simulink model "powerwindow_sl_v01"  (R2020a)
settings: Solver=ode1  StartTime=0.0  StopTime=20.0  FixedStep=0.01  RelTol=1e-3
undefined symbols (not defined in the file): auto_down_time, auto_up_time, emergency_down_time, position_endstop_top
settings Model: TunableVars=auto_down_time,auto_up_time,emergency_down_time,position_endstop_top  TunableVarsStorageClass=Auto,Auto,Auto,Auto  TunableVarsTypeQualifier=,,,  Creator=Wolfgang Meincke  LastModifiedBy=wolfgangmeincke
settings DataIOCC: LimitDataPoints=on  SaveFormat=Array  SignalLoggingSaveFormat=ModelDataLogs  ReturnWorkspaceOutputs=off
settings OptimizationCC: BlockReduction=off  BooleanDataType=off  ConditionallyExecuteInputs=off  EnableMemcpy=off  ExpressionDepthLimit=2147483647  ZeroExternalMemoryAtStartup=off  ZeroInternalMemoryAtStartup=off  InitFltsAndDblsToZero=on  NoFixptDivByZeroProtection=on  LifeSpan=1  EfficientTunableParamExpr=on
settings DebuggingCC: RTPrefix=none  SaveWithParameterizedLinksMsg=none  UnderspecifiedInitializationDetection=Classic  MergeDetectMultiDrivingBlocksExec=none  MultiTaskDSMMsg=warning  MultiTaskCondExecSysMsg=none  ParameterPrecisionLossMsg=none  FcnCallInpInsideContextMsg=warning  UnconnectedInputMsg=none  UnconnectedOutputMsg=none  StateNameClashWarn=warning  SFUnexpectedBacktrackingDiag=warning  SFNoUnconditionalDefaultTransitionDiag=warning  SFExecutionAtInitializationDiag=none  ArithmeticOperatorsInVariantConditions=warning
settings HardwareCC: ProdBitPerPointer=32  ProdBitPerSizeT=32  ProdBitPerPtrDiffT=32  ProdLargestAtomicFloat=None  ProdIntDivRoundTo=Undefined  ProdEndianess=Unspecified  ProdWordSize=32  ProdHWDeviceType=32-bit Generic
settings ModelReferenceCC: PropagateSignalLabelsOutOfModel=off
settings SFSimCC: SimUseLocalCustomCode=off  SimParseCustomCode=off  MATLABDynamicMemAlloc=off  CustomCodeUndefinedFunction=UseInterfaceOnly
settings RTWCC: SystemTargetFile=ert.tlc  GenCodeOnly=on  TemplateMakefile=ert_default_tmf  RTWUseLocalCustomCode=off
settings CodeAppCC: IgnoreCustomStorageClasses=off  ParamNamingRule=LowerCase  StateflowObjectComments=on  InternalIdentifier=Classic
settings ERTTargetCC: MultiwordLength=2048  IncludeMdlTerminateFcn=off  CombineSignalStateStructs=on  SupportAbsoluteTime=off  LogVarNameModifier=_rt  SupportNonFinite=off  SupportComplex=off  RemoveResetFunc=off  ERTCustomFileTemplate=example_file_process.tlc  ConvertIfToSwitch=off  SuppressUnreachableDefaultCases=off
settings ConfigComp: CovMetricSettings=dw  CovSaveCumulativeToWorkspaceVar=on  CovSaveSingleToWorkspaceVar=on  CovExternalEMLEnable=off

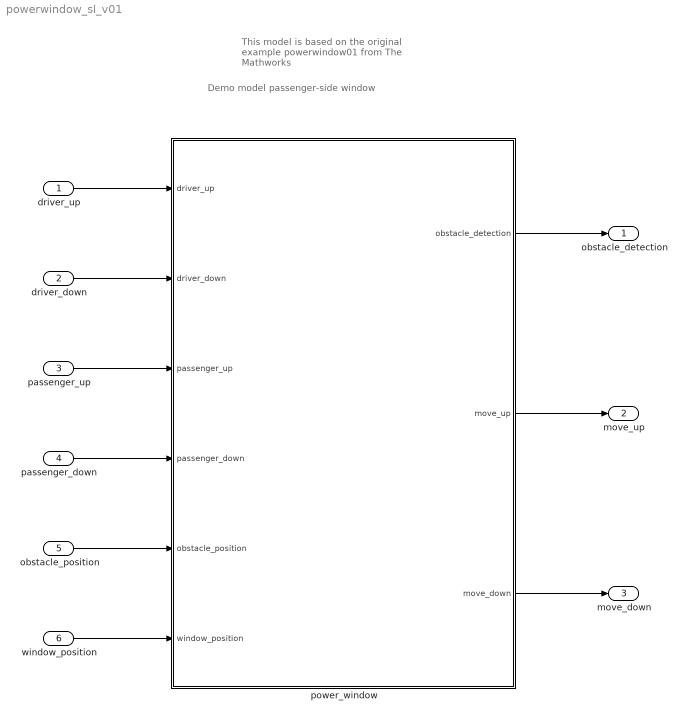
== system powerwindow_sl_v01 ==
  note: Demo model passenger-side window
  note: This model is based on the
      | original example powerwindow01
      | from The Mathworks
  driver_up : Inport  RequirementInfo={} %GIDa_c35cf34b_45f5_487d_8434_6977e2d5d2f3  OutMin=0  OutMax=1  OutDataTypeStr=boolean  PortDimensions=1
  driver_down : Inport  RequirementInfo={} %GIDa_825829a4_4c67_4036_abe4_d775b7ffbdb6  Port=2  OutMin=0  OutMax=1  OutDataTypeStr=boolean  PortDimensions=1
  passenger_up : Inport  RequirementInfo={} %GIDa_896a61d0_51a5_427e_b548_01888eb9493f  Port=3  OutMin=0  OutMax=1  OutDataTypeStr=boolean  PortDimensions=1
  passenger_down : Inport  RequirementInfo={} %GIDa_acad868a_9832_4517_80f1_eb2c424aca82  Port=4  OutMin=0  OutMax=1  OutDataTypeStr=boolean  PortDimensions=1
  obstacle_position : Inport  RequirementInfo={} %GIDa_5be180b3_640c_44df_b132_7c12c9dd4782  Port=5  OutMin=0  OutMax=0.45  OutDataTypeStr=double  PortDimensions=1
  window_position : Inport  RequirementInfo={} %GIDa_279514cf_fecf_4861_97d0_86738c273b33  Port=6  OutMin=0  OutMax=0.45  OutDataTypeStr=double  PortDimensions=1
  power_window : Subsystem
  obstacle_detection : Outport  RequirementInfo={} %GIDa_4eefd6fd_6a0d_4232_ac82_ccb47f3c36e3  OutMin=0  OutMax=1  OutDataTypeStr=boolean  PortDimensions=1
  move_up : Outport  RequirementInfo={} %GIDa_cfaa6890_1b09_43c8_9181_c9775bd2e746  Port=2  OutMin=0  OutMax=1  OutDataTypeStr=boolean  PortDimensions=1
  move_down : Outport  RequirementInfo={} %GIDa_e72b7e0a_8232_4793_901f_580fad4f0530  Port=3  OutMin=0  OutMax=1  OutDataTypeStr=boolean  PortDimensions=1
  wires:
  power_window/3(move_down) -> move_down/1
  power_window/1(obstacle_detection) -> obstacle_detection/1
  window_position/1 -> power_window/6(window_position)
  power_window/2(move_up) -> move_up/1
  driver_up/1 -> power_window/1(driver_up)
  passenger_up/1 -> power_window/3(passenger_up)
  passenger_down/1 -> power_window/4(passenger_down)
  driver_down/1 -> power_window/2(driver_down)
  obstacle_position/1 -> power_window/5(obstacle_position)

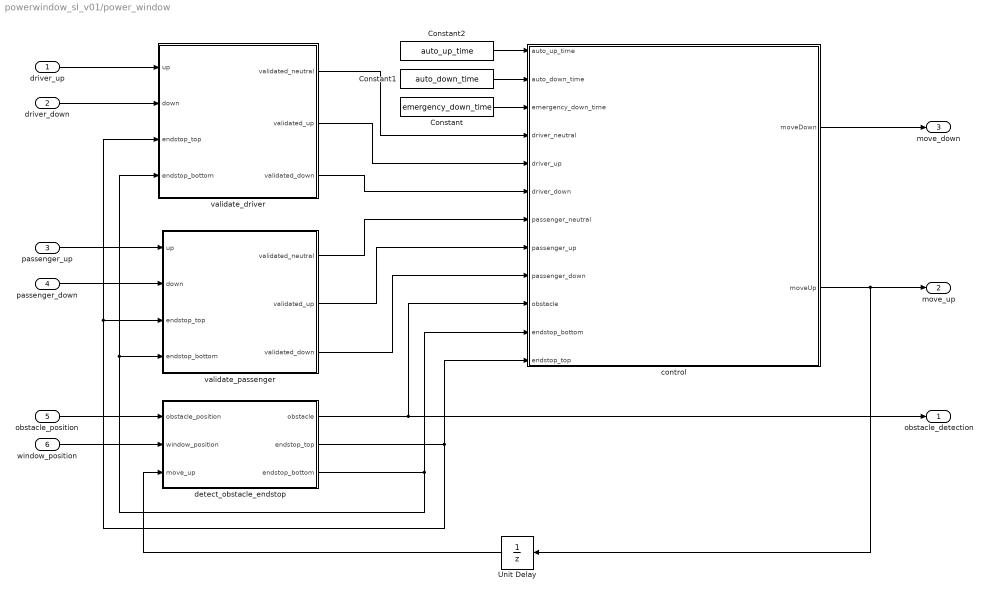
== system powerwindow_sl_v01/power_window ==
  driver_up : Inport  RequirementInfo={} %GIDa_c35cf34b_45f5_487d_8434_6977e2d5d2f3  OutMin=0  OutMax=1  OutDataTypeStr=boolean  PortDimensions=1
  driver_down : Inport  RequirementInfo={} %GIDa_825829a4_4c67_4036_abe4_d775b7ffbdb6  Port=2  OutMin=0  OutMax=1  OutDataTypeStr=boolean  PortDimensions=1
  passenger_up : Inport  RequirementInfo={} %GIDa_896a61d0_51a5_427e_b548_01888eb9493f  Port=3  OutMin=0  OutMax=1  OutDataTypeStr=boolean  PortDimensions=1
  passenger_down : Inport  RequirementInfo={} %GIDa_acad868a_9832_4517_80f1_eb2c424aca82  Port=4  OutMin=0  OutMax=1  OutDataTypeStr=boolean  PortDimensions=1
  obstacle_position : Inport  RequirementInfo={} %GIDa_5be180b3_640c_44df_b132_7c12c9dd4782  Port=5  OutMin=0  OutMax=0.45  OutDataTypeStr=double  PortDimensions=1
  window_position : Inport  RequirementInfo={} %GIDa_279514cf_fecf_4861_97d0_86738c273b33  Port=6  OutMin=0  OutMax=0.45  OutDataTypeStr=double  PortDimensions=1
  Constant : Constant  RequirementInfo={} %GIDa_9514aab4_7290_4656_a952_a9cac9bec120  Value=emergency_down_time  OutDataTypeStr=uint8
  Constant1 : Constant  RequirementInfo={} %GIDa_6c74b792_e839_4a12_ac84_86c7d570a533  Value=auto_down_time  OutDataTypeStr=uint8
  Constant2 : Constant  RequirementInfo={} %GIDa_27bbea0c_c5f9_4e52_b093_a1cd3ec1797f  Value=auto_up_time  OutDataTypeStr=uint8
  Unit Delay : UnitDelay  RequirementInfo={} %GIDa_61c3f994_badd_4b85_b577_84166d45c76a  SampleTime=-1
  control : Stateflow chart  RequirementInfo={} %GIDa_03dc6751_b1fa_4801_9ce5_d6a4ecb5c081
  detect_obstacle_endstop : Subsystem  RequirementInfo={} %GIDa_338a624e_935a_458f_b92a_1404c1b9bbb3  TreatAsAtomicUnit=on  RTWFcnName=detect_obstacle_endstop
      settings: RTWFcnNameOpts=User specified  RTWFileNameOpts=Use function name
  validate_driver : Subsystem  RequirementInfo={} %GIDa_ecdb279d_e424_4d89_b641_a52ee121c2a5  TreatAsAtomicUnit=on  RTWFcnName=validate_driver
      settings: RTWFcnNameOpts=Use subsystem name  RTWFileNameOpts=Use function name
  validate_passenger : Subsystem  RequirementInfo={} %GIDa_33b218b3_9db5_4fe6_9638_6b05429d8e58  TreatAsAtomicUnit=on  RTWFcnName=validate_passenger
      settings: RTWFcnNameOpts=User specified  RTWFileNameOpts=Use subsystem name
  obstacle_detection : Outport  RequirementInfo={} %GIDa_4eefd6fd_6a0d_4232_ac82_ccb47f3c36e3  OutMin=0  OutMax=1  OutDataTypeStr=boolean  PortDimensions=1
  move_up : Outport  RequirementInfo={} %GIDa_cfaa6890_1b09_43c8_9181_c9775bd2e746  Port=2  OutMin=0  OutMax=1  OutDataTypeStr=boolean  PortDimensions=1
  move_down : Outport  RequirementInfo={} %GIDa_e72b7e0a_8232_4793_901f_580fad4f0530  Port=3  OutMin=0  OutMax=1  OutDataTypeStr=boolean  PortDimensions=1
  wires:
  validate_passenger/2(validated_up) -> control/8(passenger_up)
  detect_obstacle_endstop/2(endstop_top) -> validate_passenger/3(endstop_top), validate_driver/3(endstop_top), control/12(endstop_top)
  validate_passenger/1(validated_neutral) -> control/7(passenger_neutral)
  detect_obstacle_endstop/1(obstacle) -> obstacle_detection/1, control/10(obstacle)
  control/2(moveUp) -> move_up/1, Unit Delay/1
  Constant/1 -> control/3(emergency_down_time)
  validate_driver/2(validated_up) -> control/5(driver_up)
  obstacle_position/1 -> detect_obstacle_endstop/1(obstacle_position)
  validate_passenger/3(validated_down) -> control/9(passenger_down)
  passenger_up/1 -> validate_passenger/1(up)
  driver_up/1 -> validate_driver/1(up)
  Constant2/1 -> control/1(auto_up_time)
  Constant1/1 -> control/2(auto_down_time)
  window_position/1 -> detect_obstacle_endstop/2(window_position)
  driver_down/1 -> validate_driver/2(down)
  detect_obstacle_endstop/3(endstop_bottom) -> validate_passenger/4(endstop_bottom), validate_driver/4(endstop_bottom), control/11(endstop_bottom)
  validate_driver/3(validated_down) -> control/6(driver_down)
  control/1(moveDown) -> move_down/1
  Unit Delay/1 -> detect_obstacle_endstop/3(move_up)
  validate_driver/1(validated_neutral) -> control/4(driver_neutral)
  passenger_down/1 -> validate_passenger/2(down)

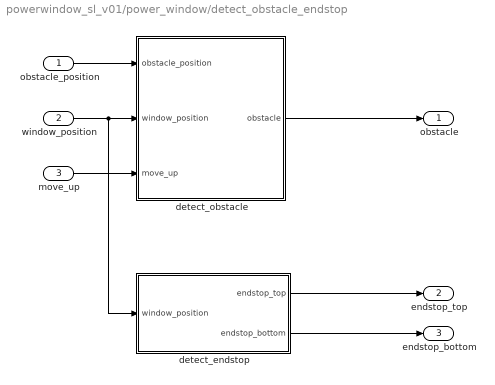
== system powerwindow_sl_v01/power_window/detect_obstacle_endstop ==
  obstacle_position : Inport  RequirementInfo={} %GIDa_129d33c9_dbad_4345_a32e_36abfffa4eb8
  window_position : Inport  RequirementInfo={} %GIDa_0a19a92c_2144_4371_9df6_11f6bf2158cd  Port=2
  move_up : Inport  RequirementInfo={} %GIDa_fb499b4a_e779_426c_9231_7bb7c4693121  Port=3
  detect_endstop : Subsystem  RequirementInfo={} %GIDa_94bbc35b_ebf0_4cc3_8650_bc7180b52bf6
  detect_obstacle : Subsystem  RequirementInfo={} %GIDa_c80b8ad7_641a_45a4_83c2_0d5a6b3dc5a0
  obstacle : Outport  RequirementInfo={} %GIDa_f8cefc1d_8d33_4143_9aaf_e393e35a8988
  endstop_top : Outport  RequirementInfo={} %GIDa_3c0c9233_5a48_409d_ac60_81b669eb4a89  Port=2
  endstop_bottom : Outport  RequirementInfo={} %GIDa_25ef007a_9840_4d98_9cf5_d35ec59ee2ed  Port=3
  wires:
  detect_endstop/2(endstop_bottom) -> endstop_bottom/1
  detect_endstop/1(endstop_top) -> endstop_top/1
  detect_obstacle/1(obstacle) -> obstacle/1
  obstacle_position/1 -> detect_obstacle/1(obstacle_position)
  window_position/1 -> detect_endstop/1(window_position), detect_obstacle/2(window_position)
  move_up/1 -> detect_obstacle/3(move_up)

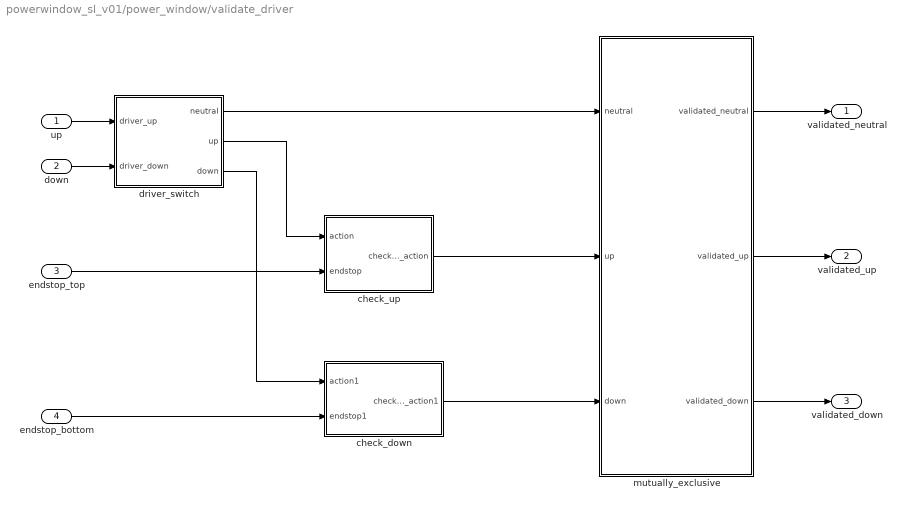
== system powerwindow_sl_v01/power_window/validate_driver ==
  up : Inport  RequirementInfo={} %GIDa_7dda3897_23eb_48f1_9817_08c06aa18141
  down : Inport  RequirementInfo={} %GIDa_9d54edea_1179_4fce_abe2_5db1acfa11b9  Port=2
  endstop_top : Inport  RequirementInfo={} %GIDa_9bd89aaf_7e8b_49dc_b3c1_497d13e079f2  Port=3
  endstop_bottom : Inport  RequirementInfo={} %GIDa_15d013e7_6fa7_49fb_8ea8_038359a3d9b6  Port=4
  check_down : Subsystem  RequirementInfo={} %GIDa_c558df2e_0968_478b_94d3_8b52e729db44
  check_up : Subsystem  RequirementInfo={} %GIDa_680f415b_674f_4667_a838_dd8371ea2197
  driver_switch : Subsystem  RequirementInfo={} %GIDa_e99d5410_be85_4670_8578_fe8e0dfb5d67
  mutually_exclusive : Subsystem  RequirementInfo={} %GIDa_d6baea27_d272_4747_8dc3_6f978df1e0c8
  validated_neutral : Outport  RequirementInfo={} %GIDa_f23c1ed9_f7cc_4416_b545_9bac5c7d020f
  validated_up : Outport  RequirementInfo={} %GIDa_9144ace2_3ce2_4646_bfcc_6ba779b8e848  Port=2
  validated_down : Outport  RequirementInfo={} %GIDa_bb002e94_52f0_4ca7_8c66_58dd2cd42898  Port=3
  wires:
  mutually_exclusive/3(validated_down) -> validated_down/1
  mutually_exclusive/2(validated_up) -> validated_up/1
  mutually_exclusive/1(validated_neutral) -> validated_neutral/1
  check_down/1(checked_action1) -> mutually_exclusive/3(down)
  check_up/1(checked_action) -> mutually_exclusive/2(up)
  driver_switch/1(neutral) -> mutually_exclusive/1(neutral)
  endstop_bottom/1 -> check_down/2(endstop1)
  endstop_top/1 -> check_up/2(endstop)
  driver_switch/3(down) -> check_down/1(action1)
  driver_switch/2(up) -> check_up/1(action)
  down/1 -> driver_switch/2(driver_down)
  up/1 -> driver_switch/1(driver_up)

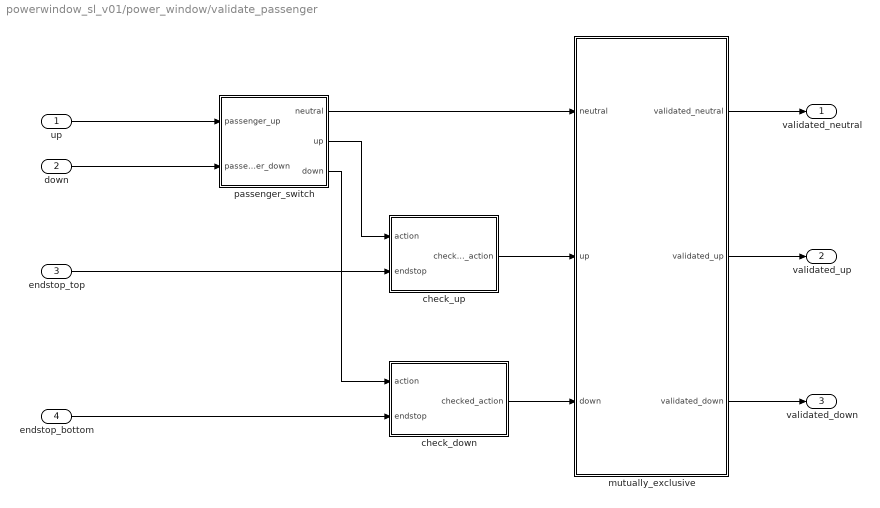
== system powerwindow_sl_v01/power_window/validate_passenger ==
  up : Inport  RequirementInfo={} %GIDa_b6408152_b334_4925_a16c_3622ca90ad97
  down : Inport  RequirementInfo={} %GIDa_df58e8e8_afe3_46fe_9c17_76802ca163b9  Port=2
  endstop_top : Inport  RequirementInfo={} %GIDa_230b0d07_e7b6_4a10_b2ed_43443fa38605  Port=3
  endstop_bottom : Inport  RequirementInfo={} %GIDa_91eacfdf_7e8f_4c54_b206_f15636a3f59e  Port=4
  check_down : Subsystem  RequirementInfo={} %GIDa_62b405b0_f053_4287_a6d2_c18d3e3b6c5b
  check_up : Subsystem  RequirementInfo={} %GIDa_92e78854_fa4d_4c59_81d3_3ea0d0c4a8a4
  mutually_exclusive : Subsystem  RequirementInfo={} %GIDa_5d841e18_2fc4_47d2_8782_e39db535edd2
  passenger_switch : Subsystem  RequirementInfo={} %GIDa_1746543f_6789_44d7_a576_254e44230f82
  validated_neutral : Outport  RequirementInfo={} %GIDa_ebd107f4_f924_4fcc_86d4_5bdc2b7613d2
  validated_up : Outport  RequirementInfo={} %GIDa_a655668a_fb1a_4125_a470_9ec06e9de417  Port=2
  validated_down : Outport  RequirementInfo={} %GIDa_d891aac2_9896_4b15_add3_213d9f963ba8  Port=3
  wires:
  mutually_exclusive/3(validated_down) -> validated_down/1
  mutually_exclusive/2(validated_up) -> validated_up/1
  mutually_exclusive/1(validated_neutral) -> validated_neutral/1
  check_down/1(checked_action) -> mutually_exclusive/3(down)
  check_up/1(checked_action) -> mutually_exclusive/2(up)
  passenger_switch/1(neutral) -> mutually_exclusive/1(neutral)
  endstop_bottom/1 -> check_down/2(endstop)
  endstop_top/1 -> check_up/2(endstop)
  passenger_switch/3(down) -> check_down/1(action)
  passenger_switch/2(up) -> check_up/1(action)
  down/1 -> passenger_switch/2(passenger_down)
  up/1 -> passenger_switch/1(passenger_up)

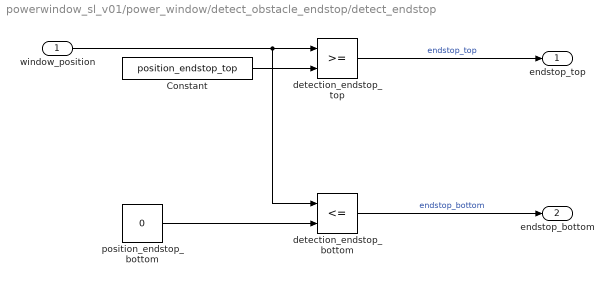
== system powerwindow_sl_v01/power_window/detect_obstacle_endstop/detect_endstop ==
  window_position : Inport  RequirementInfo={} %GIDa_dbc34208_7415_4df5_82e7_8b79bcfffe2b
  "Constant " : Constant  RequirementInfo={} %GIDa_4af3a415_bf5c_41c9_91d1_906cec003d68  Value=position_endstop_top  OutMin=0  OutMax=0.45  OutDataTypeStr=double
  detection_endstop_bottom : RelationalOperator  RequirementInfo={} %GIDa_a4cdefd8_411d_4eca_b543_424eadbfeb19  Operator=<=  OutDataTypeStr=boolean  RndMeth=Nearest
  detection_endstop_top : RelationalOperator  RequirementInfo={} %GIDa_5c8b5eae_a4e0_410d_896d_6a6cae4caa2d  OutDataTypeStr=boolean  RndMeth=Nearest
  position_endstop_bottom : Constant  RequirementInfo={} %GIDa_a8787381_1cb6_4e0b_8b4e_0c8390807a67  Value=0
  endstop_top : Outport  RequirementInfo={} %GIDa_965242d9_9a56_42ef_9050_f36606c62ef0
  endstop_bottom : Outport  RequirementInfo={} %GIDa_0bc84508_b6a5_4bab_84fe_f865e066d69b  Port=2
  wires:
  detection_endstop_bottom/1 -> endstop_bottom/1  "endstop_bottom"
  detection_endstop_top/1 -> endstop_top/1  "endstop_top"
  position_endstop_bottom/1 -> detection_endstop_bottom/2
  window_position/1 -> detection_endstop_bottom/1, detection_endstop_top/1
  "Constant "/1 -> detection_endstop_top/2

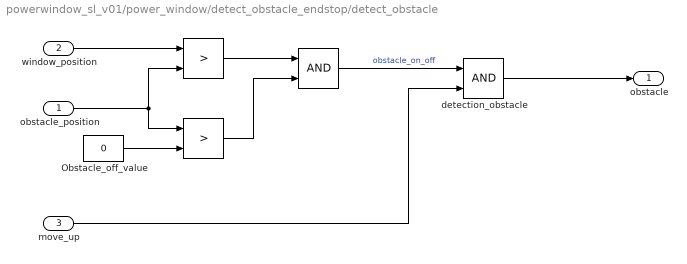
== system powerwindow_sl_v01/power_window/detect_obstacle_endstop/detect_obstacle ==
  obstacle_position : Inport  RequirementInfo={} %GIDa_a86bcfe9_2d4b_40de_8b3d_81a42c128e7b
  window_position : Inport  RequirementInfo={} %GIDa_3ff25534_ca9c_465e_9d9e_e63315ad4011  Port=2
  move_up : Inport  RequirementInfo={} %GIDa_4c7edb22_ecdc_458d_a04d_d282fa4d4cda  Port=3
  " " : Logic  RequirementInfo={} %GIDa_9a8e03f2_e713_4ca2_8608_26df95c85423  AllPortsSameDT=off  OutDataTypeStr=boolean
  "  " : RelationalOperator  RequirementInfo={} %GIDa_e32fd473_c955_4356_85a6_8629e3e025a1  Operator=>  OutDataTypeStr=boolean  RndMeth=Nearest
  "   " : RelationalOperator  RequirementInfo={} %GIDa_b41cd641_ca58_444b_bb87_9c7524fc2f1e  Operator=>  OutDataTypeStr=boolean  RndMeth=Nearest
  Obstacle_off_value : Constant  RequirementInfo={} %GIDa_9c20d162_dea6_4c97_9178_9dd066c384fc  Value=0
  detection_obstacle : Logic  RequirementInfo={} %GIDa_a4339f7b_ead1_49ab_bc60_e53143b57e09  AllPortsSameDT=off  OutDataTypeStr=boolean
  obstacle : Outport  RequirementInfo={} %GIDa_42986494_1328_4df5_b7f7_1e70c8f47b53
  wires:
  Obstacle_off_value/1 -> "   "/2
  obstacle_position/1 -> "  "/2, "   "/1
  "   "/1 -> " "/2
  move_up/1 -> detection_obstacle/2
  " "/1 -> detection_obstacle/1  "obstacle_on_off"
  "  "/1 -> " "/1
  window_position/1 -> "  "/1
  detection_obstacle/1 -> obstacle/1

== system powerwindow_sl_v01/power_window/validate_driver/check_down ==
  action1 : Inport  RequirementInfo={} %GIDa_bfe33c50_b0b7_4229_9a33_0a89dd964ee4
  endstop1 : Inport  RequirementInfo={} %GIDa_3bef5000_1405_47aa_b5ec_d4618ab525dc  Port=2
  Terminator : Terminator
  checked_action1 : Outport  RequirementInfo={} %GIDa_9b4768a3_2f87_4844_a7eb_26344070ec4c
  wires:
  action1/1 -> checked_action1/1
  endstop1/1 -> Terminator/1

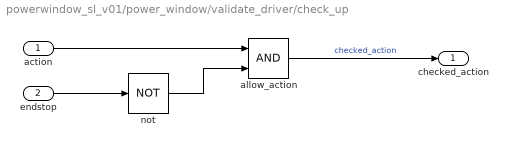
== system powerwindow_sl_v01/power_window/validate_driver/check_up ==
  action : Inport  RequirementInfo={} %GIDa_230d8a4d_0933_44fe_9611_b9b5e97283aa
  endstop : Inport  RequirementInfo={} %GIDa_66508a74_de66_457c_af9b_58ca17601a68  Port=2
  allow_action : Logic  RequirementInfo={} %GIDa_c19d02dd_ee13_48de_a1d1_6b21862bf281  AllPortsSameDT=off  OutDataTypeStr=boolean
  not : Logic  RequirementInfo={} %GIDa_d5e73d0e_c736_4c2c_b977_57a558d08b37  Operator=NOT  Inputs=1  AllPortsSameDT=off  OutDataTypeStr=boolean
  checked_action : Outport  RequirementInfo={} %GIDa_ff7fcc47_378b_4377_8913_af8241850286
  wires:
  not/1 -> allow_action/2
  endstop/1 -> not/1
  action/1 -> allow_action/1
  allow_action/1 -> checked_action/1  "checked_action"

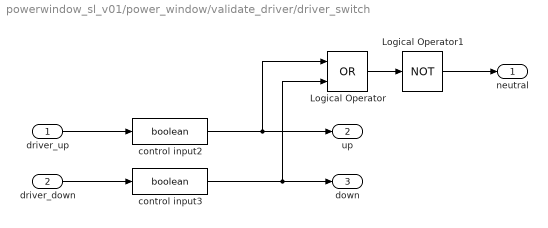
== system powerwindow_sl_v01/power_window/validate_driver/driver_switch ==
  driver_up : Inport  RequirementInfo={} %GIDa_7854071d_2c86_4c0b_ab89_d6784a1228c6
  driver_down : Inport  RequirementInfo={} %GIDa_bb711ebe_242d_4f7e_88e1_00cfa0b4d3f9  Port=2
  Logical Operator : Logic  RequirementInfo={} %GIDa_d6c2960b_addd_4a1a_812f_73adf7540583  Operator=OR  AllPortsSameDT=off  OutDataTypeStr=boolean
  Logical Operator1 : Logic  RequirementInfo={} %GIDa_8834cba1_a9e6_4b65_841d_1b2357c8c5c2  Operator=NOT  Inputs=1  AllPortsSameDT=off  OutDataTypeStr=boolean
  control input2 : DataTypeConversion  RequirementInfo={} %GIDa_2895f3c2_8950_49a6_830a_3b04837805c2  OutDataTypeStr=boolean  SaturateOnIntegerOverflow=on  RndMeth=Zero
  control input3 : DataTypeConversion  RequirementInfo={} %GIDa_d53e04af_1d89_4524_a64c_0a4214a606b4  OutDataTypeStr=boolean  SaturateOnIntegerOverflow=on  RndMeth=Zero
  neutral : Outport  RequirementInfo={} %GIDa_598fa772_5b98_4d33_9205_b8bb5679c75b
  up : Outport  RequirementInfo={} %GIDa_11133d49_a9d8_488f_9ba5_efdd3785f25a  Port=2
  down : Outport  RequirementInfo={} %GIDa_36307aa9_1d87_4893_a1a9_7f8ce36e7330  Port=3
  wires:
  Logical Operator1/1 -> neutral/1
  Logical Operator/1 -> Logical Operator1/1
  control input3/1 -> Logical Operator/2, down/1
  control input2/1 -> Logical Operator/1, up/1
  driver_down/1 -> control input3/1
  driver_up/1 -> control input2/1

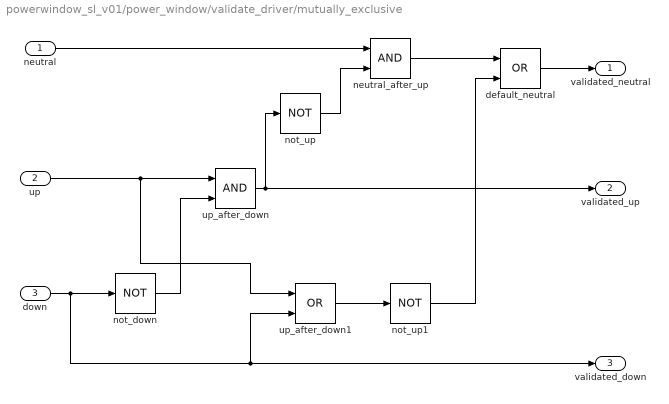
== system powerwindow_sl_v01/power_window/validate_driver/mutually_exclusive ==
  neutral : Inport  RequirementInfo={} %GIDa_a03c26c0_75be_4e7b_aebf_4ee68fef49d5
  up : Inport  RequirementInfo={} %GIDa_c015af08_de8a_43c0_8aeb_e7ba93c2f7b3  Port=2
  down : Inport  RequirementInfo={} %GIDa_e3cb6b32_180a_4bbe_a210_7c7014f55eff  Port=3
  default_neutral : Logic  RequirementInfo={} %GIDa_e3cd5f36_2c72_43b0_af8f_c2ba3eb25f44  Operator=OR  AllPortsSameDT=off  OutDataTypeStr=boolean
  neutral_after_up : Logic  RequirementInfo={} %GIDa_d6ca6eb7_ba2e_48b6_ad53_6af510ed347f  AllPortsSameDT=off  OutDataTypeStr=boolean
  not_down : Logic  RequirementInfo={} %GIDa_71cef795_930c_4d49_b324_e926110cc8ee  Operator=NOT  Inputs=1  AllPortsSameDT=off  OutDataTypeStr=boolean
  not_up : Logic  RequirementInfo={} %GIDa_66ad6d87_a5f8_459c_9da3_faf5e8dbdf35  Operator=NOT  Inputs=1  AllPortsSameDT=off  OutDataTypeStr=boolean
  not_up1 : Logic  RequirementInfo={} %GIDa_548b9df8_c35a_4dd3_9653_ed9c05316059  Operator=NOT  Inputs=1  AllPortsSameDT=off  OutDataTypeStr=boolean
  up_after_down : Logic  RequirementInfo={} %GIDa_60f9e124_17bc_41bc_86c8_4d7d48148db4  AllPortsSameDT=off  OutDataTypeStr=boolean
  up_after_down1 : Logic  RequirementInfo={} %GIDa_cf8a62dc_6640_429b_b212_174f06d78f92  Operator=OR  AllPortsSameDT=off  OutDataTypeStr=boolean
  validated_neutral : Outport  RequirementInfo={} %GIDa_434f7c26_4302_46cf_a0ac_5e8349f5a85a
  validated_up : Outport  RequirementInfo={} %GIDa_5a7209c8_9501_4720_a7b3_09da770970d2  Port=2
  validated_down : Outport  RequirementInfo={} %GIDa_ccca83ea_3e87_429a_969e_1868ccac4351  Port=3
  wires:
  default_neutral/1 -> validated_neutral/1
  neutral_after_up/1 -> default_neutral/1
  not_up1/1 -> default_neutral/2
  up_after_down1/1 -> not_up1/1
  not_down/1 -> up_after_down/2
  down/1 -> up_after_down1/2, validated_down/1, not_down/1
  up/1 -> up_after_down1/1, up_after_down/1
  up_after_down/1 -> not_up/1, validated_up/1
  not_up/1 -> neutral_after_up/2
  neutral/1 -> neutral_after_up/1

== system powerwindow_sl_v01/power_window/validate_passenger/check_down ==
  action : Inport  RequirementInfo={} %GIDa_ca512674_cbe4_48ba_9017_69e0f816f711
  endstop : Inport  RequirementInfo={} %GIDa_59664dfc_9454_41cf_927b_a889b06514c8  Port=2
  allow_action : Logic  RequirementInfo={} %GIDa_6d61b7cc_cf4f_459c_8f84_8bb0cf779dee  AllPortsSameDT=off  OutDataTypeStr=boolean
  not : Logic  RequirementInfo={} %GIDa_75feb0d0_87dd_4abc_903e_36f510d82096  Operator=NOT  Inputs=1  AllPortsSameDT=off  OutDataTypeStr=boolean
  checked_action : Outport  RequirementInfo={} %GIDa_6a46bd9b_176e_4e3e_a6a8_fff5e40471e2
  wires:
  action/1 -> allow_action/1
  not/1 -> allow_action/2
  allow_action/1 -> checked_action/1  "checked_action"
  endstop/1 -> not/1

== system powerwindow_sl_v01/power_window/validate_passenger/check_up ==
  action : Inport  RequirementInfo={} %GIDa_dc7fa4e4_fe57_40ae_a062_8dffeb9176be
  endstop : Inport  RequirementInfo={} %GIDa_5af3944e_bdc7_478a_9674_1af1981846f4  Port=2
  allow_action : Logic  RequirementInfo={} %GIDa_96999e18_96cd_470f_ae60_b66afebaee89  AllPortsSameDT=off  OutDataTypeStr=boolean
  not : Logic  RequirementInfo={} %GIDa_a0499630_f6e4_41e6_ae99_6236f2ab45db  Operator=NOT  Inputs=1  AllPortsSameDT=off  OutDataTypeStr=boolean
  checked_action : Outport  RequirementInfo={} %GIDa_8039e34e_7a32_4eab_98be_7588d21475d6
  wires:
  not/1 -> allow_action/2
  endstop/1 -> not/1
  action/1 -> allow_action/1
  allow_action/1 -> checked_action/1  "checked_action"

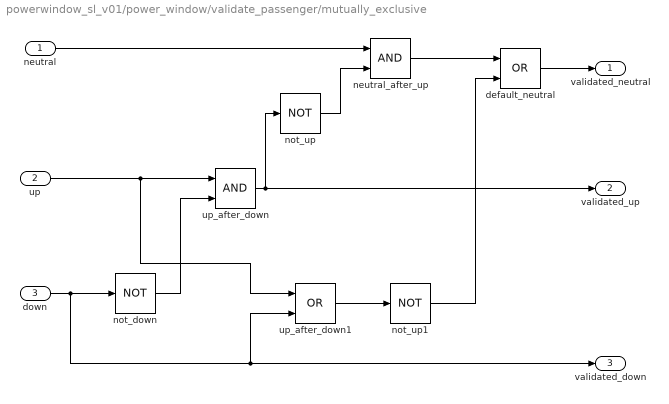
== system powerwindow_sl_v01/power_window/validate_passenger/mutually_exclusive ==
  neutral : Inport  RequirementInfo={} %GIDa_8f003c53_0f06_402c_bf11_e1dae5ac4ba2
  up : Inport  RequirementInfo={} %GIDa_13e7cfed_65e8_4439_989f_1cf26328e825  Port=2
  down : Inport  RequirementInfo={} %GIDa_b18b33e4_0100_4836_9df2_c076b889bc83  Port=3
  default_neutral : Logic  RequirementInfo={} %GIDa_721e8f87_b194_487a_970a_3a929a776efa  Operator=OR  AllPortsSameDT=off  OutDataTypeStr=boolean
  neutral_after_up : Logic  RequirementInfo={} %GIDa_099c4db0_1ced_407c_9a11_52cdc433151a  AllPortsSameDT=off  OutDataTypeStr=boolean
  not_down : Logic  RequirementInfo={} %GIDa_21e7df57_4079_420c_aa24_638c8886d47b  Operator=NOT  Inputs=1  AllPortsSameDT=off  OutDataTypeStr=boolean
  not_up : Logic  RequirementInfo={} %GIDa_ba891d16_2ab0_4455_8efb_8452a25ddce4  Operator=NOT  Inputs=1  AllPortsSameDT=off  OutDataTypeStr=boolean
  not_up1 : Logic  RequirementInfo={} %GIDa_d7755c1f_7020_4217_ac48_627cd233c0c5  Operator=NOT  Inputs=1  AllPortsSameDT=off  OutDataTypeStr=boolean
  up_after_down : Logic  RequirementInfo={} %GIDa_6c1a5302_81e3_4f31_8645_f01e65565135  AllPortsSameDT=off  OutDataTypeStr=boolean
  up_after_down1 : Logic  RequirementInfo={} %GIDa_68cb3128_3b52_420a_b6c5_4a84693a377b  Operator=OR  AllPortsSameDT=off  OutDataTypeStr=boolean
  validated_neutral : Outport  RequirementInfo={} %GIDa_49ff77a4_e54e_4e57_8264_91fcfa71c2f8
  validated_up : Outport  RequirementInfo={} %GIDa_c13404c1_0905_4a17_a186_e38525a7269f  Port=2
  validated_down : Outport  RequirementInfo={} %GIDa_f8e3c94c_9fee_405f_8ae0_09bb929cc26c  Port=3
  wires:
  default_neutral/1 -> validated_neutral/1
  neutral_after_up/1 -> default_neutral/1
  not_up1/1 -> default_neutral/2
  up_after_down1/1 -> not_up1/1
  not_down/1 -> up_after_down/2
  down/1 -> up_after_down1/2, validated_down/1, not_down/1
  up/1 -> up_after_down1/1, up_after_down/1
  up_after_down/1 -> not_up/1, validated_up/1
  not_up/1 -> neutral_after_up/2
  neutral/1 -> neutral_after_up/1

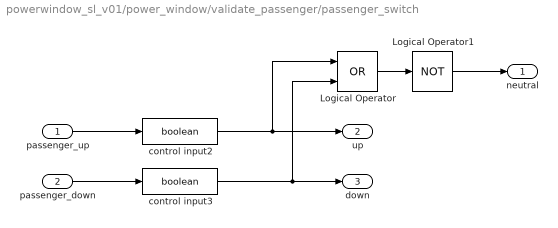
== system powerwindow_sl_v01/power_window/validate_passenger/passenger_switch ==
  passenger_up : Inport  RequirementInfo={} %GIDa_61b4d6eb_b343_41f6_8a80_dcc5328050d4
  passenger_down : Inport  RequirementInfo={} %GIDa_159ae53f_aacb_4aa9_ab9b_f7d3b5ed93b6  Port=2
  Logical Operator : Logic  RequirementInfo={} %GIDa_7d1f1e29_2525_49a5_8297_8d1857c67a70  Operator=OR  AllPortsSameDT=off  OutDataTypeStr=boolean
  Logical Operator1 : Logic  RequirementInfo={} %GIDa_c67391d6_db29_412d_911b_665d5b7f1999  Operator=NOT  Inputs=1  AllPortsSameDT=off  OutDataTypeStr=boolean
  control input2 : DataTypeConversion  RequirementInfo={} %GIDa_15e65c4a_7f2f_4a03_ad86_98d237be47e6  OutDataTypeStr=boolean  SaturateOnIntegerOverflow=on  RndMeth=Zero
  control input3 : DataTypeConversion  RequirementInfo={} %GIDa_44021398_892f_4942_b995_99cb371ef146  OutDataTypeStr=boolean  SaturateOnIntegerOverflow=on  RndMeth=Zero
  neutral : Outport  RequirementInfo={} %GIDa_82178efc_15f5_4b92_893f_50e480dd7654
  up : Outport  RequirementInfo={} %GIDa_9ba8bbc2_f4d4_4c2a_a343_4354814556d4  Port=2
  down : Outport  RequirementInfo={} %GIDa_e2954a87_897d_46fb_be12_5a148406f165  Port=3
  wires:
  Logical Operator1/1 -> neutral/1
  Logical Operator/1 -> Logical Operator1/1
  control input3/1 -> Logical Operator/2, down/1
  control input2/1 -> Logical Operator/1, up/1
  passenger_down/1 -> control input3/1
  passenger_up/1 -> control input2/1

== stateflow chart powerwindow_sl_v01/power_window/control ==
  state safe
    state driverNeutral
      entry:
      moveUp = 0;
      moveDown = 0;
      state passengerneutral
        entry:
        moveUp = 0;
        moveDown = 0;
      state passengerDown
        entry: moveDown = 1;
        exit:   moveDown = 0;
        state iniPassengerDown
        state passengerDown
        state autoPassengerDown
        iniPassengerDown -> (junction 14) : after(auto_down_time,tick)
        (junction 14) -> safe.driverNeutral.passengerDown.passengerDown [order 2]
        (junction 14) -> autoPassengerDown [order 1] : [passenger_neutral]
      state passengerUp
        entry: moveUp = 1;
        exit: moveUp = 0;
        state iniPassengerUp
        state PassengerUp
        state autoPassengerUp
        iniPassengerUp -> (junction 29) : after(auto_up_time,tick)
        (junction 29) -> PassengerUp [order 2]
        (junction 29) -> autoPassengerUp [order 1] : [passenger_neutral]
      (default) -> passengerneutral
      passengerneutral -> iniPassengerUp [order 1] : [passenger_up]
      passengerneutral -> iniPassengerDown [order 2] : [passenger_down]
      safe.driverNeutral.passengerDown.passengerDown -> passengerneutral : [passenger_neutral]
      PassengerUp -> passengerneutral : [passenger_neutral]
      safe.driverNeutral.passengerDown -> passengerneutral [order 1] : [endstop_bottom]
      passengerUp -> passengerneutral [order 2] : [endstop_top]
      safe.driverNeutral.passengerDown -> PassengerUp [order 2] : [passenger_up]
      passengerUp -> safe.driverNeutral.passengerDown.passengerDown [order 1] : [passenger_down]
    state driverUp
      entry: moveUp = 1;
      exit: moveUp = 0;
      state iniDriverUp
      state DriverUp
      state autoDriverUp
      iniDriverUp -> (junction 55) : after(auto_up_time,tick)
      (junction 55) -> DriverUp [order 2]
      (junction 55) -> autoDriverUp [order 1] : [driver_neutral]
    state driverDown
      entry: moveDown = 1;
      exit: moveDown = 0;
      state iniDriverDown
      state DriverDown
      state autoDriverDown
      iniDriverDown -> (junction 44) : after(auto_down_time,tick)
      (junction 44) -> DriverDown [order 2]
      (junction 44) -> autoDriverDown [order 1] : [driver_neutral]
    (default) -> driverNeutral
    driverNeutral -> iniDriverDown [order 2] : [driver_down]
    DriverDown -> driverNeutral : [driver_neutral]
    driverDown -> driverNeutral [order 1] : [endstop_bottom]
    DriverUp -> driverNeutral : [driver_neutral]
    driverUp -> driverNeutral [order 2] : [endstop_top]
    driverNeutral -> iniDriverUp [order 1] : [driver_up]
    driverDown -> DriverUp [order 2] : [driver_up]
    driverUp -> DriverDown [order 1] : [driver_down]
  state emergencyDown
    entry:
    moveUp = 0;
    moveDown = 1;
  emergencyDown -> passengerneutral : [endstop_bottom | after(emergency_down_time,tick)]
  (default) -> safe
  driverNeutral -> emergencyDown [order 3] : [obstacle]
  data: auto_up_time input; auto_down_time input; emergency_down_time input; driver_neutral input; driver_up input; driver_down input; passenger_neutral input; passenger_up input; passenger_down input; obstacle input; endstop_bottom input; endstop_top input; moveDown output; moveUp output
  data driver_neutral settings: description=$TL$ type=Bool; $TL$
  data driver_up settings: description=$TL$ type=Bool; $TL$
  data driver_down settings: description=$TL$ type=Bool; $TL$
  data passenger_neutral settings: description=$TL$ type=Bool; $TL$
  data passenger_up settings: description=$TL$ type=Bool; $TL$
  data passenger_down settings: description=$TL$ type=Bool; $TL$
  data obstacle settings: description=$TL$ type=Bool; $TL$
  data endstop_bottom settings: description=$TL$ type=Bool; $TL$
  data endstop_top settings: description=$TL$ type=Bool; $TL$
